simulink model "ifelse_mdl"  (Simulink 7.9)
settings: Solver=ode45  StartTime=0.0  StopTime=20.0  RelTol=1e-3
settings Model: Creator=hujh  LastModifiedBy=hujh

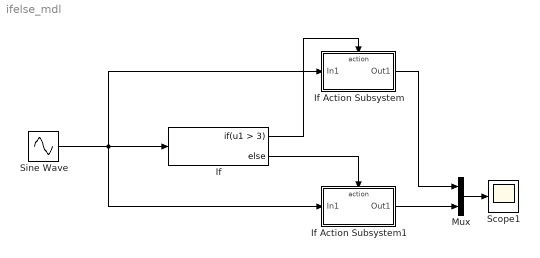
== system ifelse_mdl ==
  If : If  IfExpression=u1 > 3
  If Action Subsystem : Subsystem  TreatAsAtomicUnit=on
  If Action Subsystem1 : Subsystem  TreatAsAtomicUnit=on
  Mux : Mux  Inputs=2
  Scope1 : Scope
  Sine Wave : Sin  Amplitude=5  SampleTime=0
  wires:
  Sine Wave/1 -> If/1, If Action Subsystem/1(In1), If Action Subsystem1/1(In1)
  If Action Subsystem1/1(Out1) -> Mux/2
  If Action Subsystem/1(Out1) -> Mux/1
  If/1 -> If Action Subsystem/Action
  If/2 -> If Action Subsystem1/Action
  Mux/1 -> Scope1/1

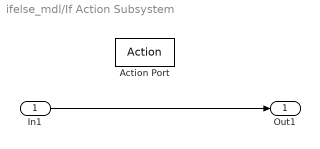
== system ifelse_mdl/If Action Subsystem ==
  In1 : Inport
  Action Port : ActionPort  ActionType=then
  Out1 : Outport
  wires:
  In1/1 -> Out1/1

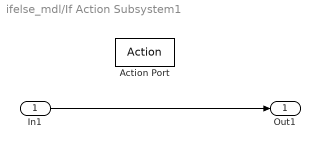
== system ifelse_mdl/If Action Subsystem1 ==
  In1 : Inport
  Action Port : ActionPort  ActionType=else
  Out1 : Outport
  wires:
  In1/1 -> Out1/1
